simulink model "t1_sim"  (Simulink 7.3)
settings: Solver=ode45  StartTime=0.0  StopTime=5  RelTol=1e-3
values from neighbouring files (symbols this model uses):
  B = 5    [t1.m]
  gc = tf([354.25 88.4],[1 0])    [t1.m]
  K = 50    [t1.m]
  M = 1    [t1.m]
  Ts = .02    (= 0.02)    [t1.m]
settings Model: Creator=arash  LastModifiedBy=arash

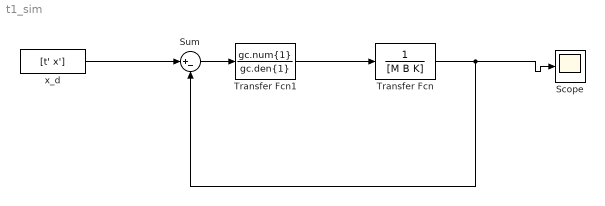
== system t1_sim ==
  Scope : Scope
  Sum : Sum  Inputs=|+-  OutDataType=fixdt(1, 16)  OutScaling=2^0
  Transfer Fcn : TransferFcn  Numerator=1  Denominator=[M B K]
  Transfer Fcn1 : TransferFcn  Numerator=gc.num{1}  Denominator=gc.den{1}
  x_d : FromWorkspace  VariableName=[t' x']  SampleTime=Ts
  wires:
  Transfer Fcn/1 -> Scope/1, Sum/2
  Transfer Fcn1/1 -> Transfer Fcn/1
  Sum/1 -> Transfer Fcn1/1
  x_d/1 -> Sum/1
